simulink model "buck_lqr_4"  (R2020a)
settings: Solver=VariableStepAuto  StartTime=0.0  StopTime=0.1  RelTol=1e-3
libraries: powerlib x12, powerlib_meascontrol x1
settings Model: Creator=ayanc  LastModifiedBy=ayanc

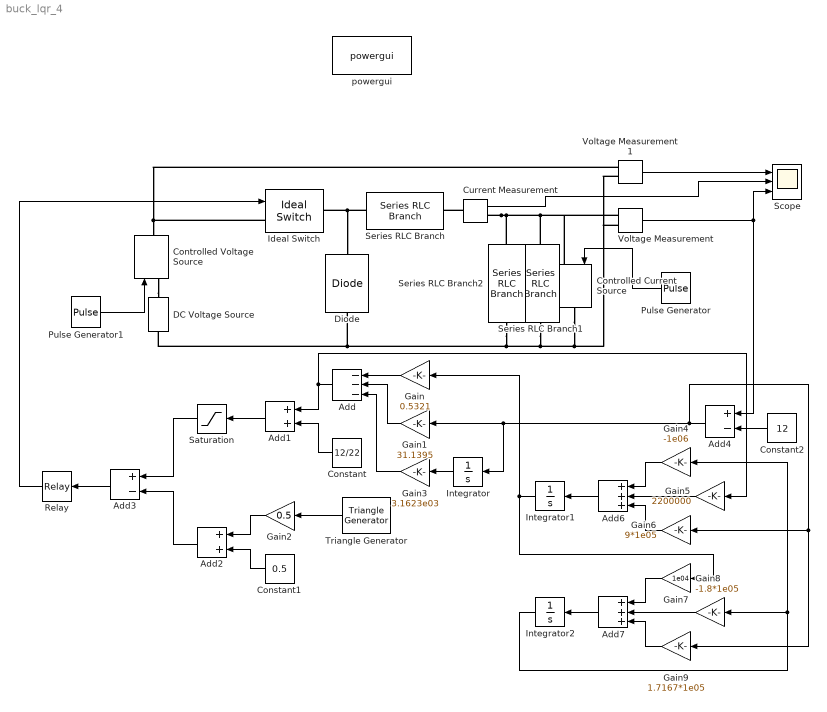
== system buck_lqr_4 ==
  Add : Sum  Inputs=---
  Add1 : Sum
  Add2 : Sum
  Add3 : Sum  Inputs=+-
  Add4 : Sum  Inputs=+-
  Add6 : Sum  Inputs=+++
  Add7 : Sum  Inputs=+++
  Constant : Constant  Value=12/22
  Constant1 : Constant  Value=0.5
  Constant2 : Constant  Value=12
  Controlled Current Source : powerlib/Electrical Sources/Controlled Current Source  Initialize=on  Source_Type=DC  Amplitude=0  Phase=0  Frequency=0  Measurements=None
  Controlled Voltage Source : powerlib/Electrical Sources/Controlled Voltage Source  Initialize=on  Source_Type=DC  Amplitude=0  Phase=0  Frequency=0  Measurements=None
  Current Measurement : powerlib/Measurements/Current Measurement  PhasorSimulation=off  OutputType=Complex  PSBequivalent=0
  DC Voltage Source : powerlib/Electrical Sources/DC Voltage Source  Amplitude=22  Measurements=None
  Diode : powerlib/Power Electronics/Diode  Ron=0  Lon=0  Vf=0  IC=0  UseSnubber=0  Rs=inf  Cs=0  Measurements=off
  Gain : Gain  Gain=0.5321
  Gain1 : Gain  Gain=31.1395
  Gain2 : Gain  Gain=0.5
  Gain3 : Gain  Gain=3.1623e03
  Gain4 : Gain  Gain=-1e06
  Gain5 : Gain  Gain=2200000
  Gain6 : Gain  Gain=9*1e05
  Gain7 : Gain  Gain=1e04
  Gain8 : Gain  Gain=-1.8*1e05
  Gain9 : Gain  Gain=1.7167*1e05
  Ideal Switch : powerlib/Power Electronics/Ideal Switch  Ron=0  Lon=0  IC=0  Rs=inf  Cs=inf  Measurements=off
  Integrator : Integrator
  Integrator1 : Integrator
  Integrator2 : Integrator
  Pulse Generator : DiscretePulseGenerator  PulseType=Time based  Amplitude=5  Period=0.04  PulseWidth=50  PhaseDelay=0.01
  Pulse Generator1 : DiscretePulseGenerator  PulseType=Time based  Amplitude=5  Period=0.04  PulseWidth=50  PhaseDelay=0.05
  Relay : Relay
  Saturation : Saturate  UpperLimit=1  LowerLimit=0  ZeroCross=off
  Scope : Scope  NumInputPorts=3
  Series RLC Branch : powerlib/Elements/Series RLC Branch  LConnTagsString=__new0  RConnTagsString=__new0  BranchType=L  Resistance=1  Inductance=10e-06  SetiL0=off  InitialCurrent=0  Capacitance=1e-6  Setx0=off  InitialVoltage=0  Measurements=None
  Series RLC Branch1 : powerlib/Elements/Series RLC Branch  LConnTagsString=__new0  RConnTagsString=__new0  BranchType=R  Resistance=1.2  Inductance=1e-3  SetiL0=off  InitialCurrent=0  Capacitance=1e-6  Setx0=off  InitialVoltage=0  Measurements=None
  Series RLC Branch2 : powerlib/Elements/Series RLC Branch  LConnTagsString=__new0  RConnTagsString=__new0  BranchType=C  Resistance=1  Inductance=1e-3  SetiL0=off  InitialCurrent=0  Capacitance=100e-06  Setx0=off  InitialVoltage=0  Measurements=None
  Triangle Generator : powerlib_meascontrol/Pulse & Signal Generators/Triangle Generator  Freq=500e3  Phase=90  Ts=0
  Voltage Measurement : powerlib/Measurements/Voltage Measurement  PhasorSimulation=off  OutputType=Complex  PSBequivalent=0
  Voltage Measurement1 : powerlib/Measurements/Voltage Measurement  PhasorSimulation=off  OutputType=Complex  PSBequivalent=0
  powergui : powerlib/powergui  Priority=1  SimulationMode=Continuous  SampleTime=50e-6  frequency=60  Iterations=50  frequencyindice=0  Pbase=100e6  ErrMax=1e-4  UnitsV=kV  UnitsW=MW  buscounter=0  FunctionMessages=off  echomessages=off  EnableUseOfTLC=off  CurrentSourceSwitches=off  DisableSnubberDevices=off  DisableRonSwitches=off  DisableVfSwitches=off  DisplayEquations=off  AutomaticDiscreteSolvers=off  SolverType=Tustin/Backward Euler (TBE)  Interpol=off  ExternalGateDelay=off  methode=off  Ts=100  x0status=blocks  SPID=on  SwTol=0  HookPort=off  NonlinearTolerance=1e-4  nMaxIteration=100  ContinueOnMaxIteration=off  RestoreLinks=warning  ResistiveCurrentMeasurement=off  Frange=[0:2:500]  Ylog=off  Xlog=on  ShowGrid=off  save=off  variable=ZData  structure=0  ZoomFFT=off  StartTime=0.0  cycles=1  DisplayStyle=1  fundamental=60  FreqAxis=off  MaxFrequency=1000  frequencyindicesteady=1  RmsSteady=1  display=off
  wires:
  Add2/1 -> Add3/2
  Gain3/1 -> Add/3
  Gain1/1 -> Add/2
  Gain2/1 -> Add2/1
  Constant/1 -> Add1/2
  Saturation/1 -> Add3/1
  Add1/1 -> Saturation/1
  Integrator/1 -> Gain3/1
  Voltage Measurement/1 -> Scope/3, Add4/1
  Add/1 -> Gain5/1, Add1/1
  Relay/1 -> Ideal Switch/1
  Triangle Generator/1 -> Gain2/1
  Add3/1 -> Relay/1
  Constant1/1 -> Add2/2
  Gain/1 -> Add/1
  Gain8/1 -> Add7/2
  Add6/1 -> Integrator1/1
  Gain9/1 -> Add7/3
  Gain7/1 -> Add7/1
  Add4/1 -> Integrator/1, Gain1/1, Gain9/1, Gain6/1
  Gain6/1 -> Add6/3
  Gain4/1 -> Add6/1
  Gain5/1 -> Add6/2
  Integrator2/1 -> Gain8/1, Gain4/1
  Integrator1/1 -> Gain/1, Gain7/1
  Constant2/1 -> Add4/2
  Add7/1 -> Integrator2/1
  Pulse Generator1/1 -> Controlled Voltage Source/1
  Voltage Measurement1/1 -> Scope/1
  Current Measurement/1 -> Scope/2
  Pulse Generator/1 -> Controlled Current Source/1
  connections:
  Series RLC Branch2/RConn1 -- Voltage Measurement1/LConn2 -- Voltage Measurement/LConn2 -- Controlled Current Source/RConn1 -- Series RLC Branch1/RConn1 -- Diode/LConn1 -- DC Voltage Source/LConn1
  Current Measurement/RConn1 -- Series RLC Branch2/LConn1 -- Controlled Current Source/LConn1 -- Voltage Measurement/LConn1 -- Series RLC Branch1/LConn1
  Series RLC Branch/LConn1 -- Ideal Switch/RConn1 -- Diode/RConn1
  Current Measurement/LConn1 -- Series RLC Branch/RConn1
  Controlled Voltage Source/LConn1 -- DC Voltage Source/RConn1
  Ideal Switch/LConn1 -- Voltage Measurement1/LConn1 -- Controlled Voltage Source/RConn1
